simulink model "wingrockCustom"  (R2025b)
settings: Solver=VariableStepAuto  StartTime=0.0  StopTime=Tf  RelTol=1e-3
undefined symbols (not defined in the file): A, B
libraries: slctrl_adaptive x1
settings Model: Creator=The MathWorks, Inc.  LastModifiedBy=The MathWorks, Inc.
settings SolverCC: MaxZcPerStep=1.0
settings DebuggingCC: UnconnectedInputMsg=warning  UnconnectedOutputMsg=warning  UnconnectedLineMsg=warning
settings ModelReferenceCC: EnableRefExpFcnMdlSchedulingChecks=on
settings RTWCC: GPUComputeCapability=3.5  DLArmComputeVersion=19.05

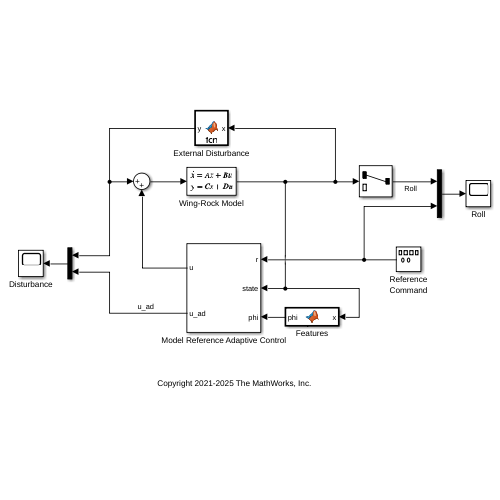
[thumbnail: Simulink's stored preview of the top-level diagram]
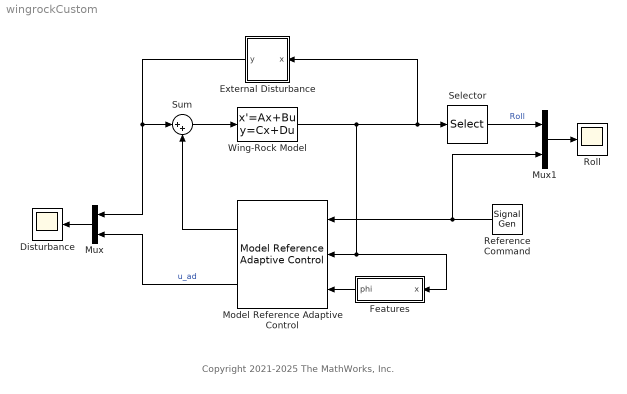
== system wingrockCustom ==
  note: Copyright 2021-2025 The MathWorks, Inc.
  Disturbance : Scope
      settings: ActiveDisplayYMinimum=-4.33702  ActiveDisplayYMaximum=6.96023
  External Disturbance : MATLAB Function  TreatAsAtomicUnit=on
  Features : MATLAB Function  TreatAsAtomicUnit=on
  Model Reference Adaptive Control : slctrl_adaptive/Model Reference Adaptive Control  selectType=Direct  A=A  B=B  Ahat=0  ALrEnable=on  gamma_a=1  ALrEnableMod=on  Bhat=1  BLrEnable=on  gamma_b=1  BLrEnableMod=on  externalKtauEnable=off  k_tau=-1  estParamOutput=off  Am=Am  Bm=Bm  kx=Kx  FBLrEnable=off  gamma_kx=1  FBLrEnableMod=on  kr=Kr  FFLrEnable=off  gamma_kr=1  FFLrEnableMod=on  AdaptEnable=on  gamma=gamma_w  WLrEnableMod=off  Q=Q  FeatureTypeOptions=Use External Source for Feature  shlHiddenLayerSize=10  gamma_V=0.1  nCen=N  cSpanMin=cen_min  cSpanMax=cen_max  cSig=bandwidth  adaptiveCntrlOutport=on  modChoice=None  sigma_val=0.1  DiscreteEnable=off  Ts=0.05  IntegrationMethods=Forward Euler
      settings: LibrarySourceBlock=slctrlblks/Adaptive Control/Model Reference Adaptive Control
  Mux : Mux  Inputs=2
  Mux1 : Mux  Inputs=2
  Reference Command : SignalGenerator  WaveForm=square  Frequency=0.5  Units=rad/sec
  Roll : Scope
      settings: ActiveDisplayYMinimum=-1.67014  ActiveDisplayYMaximum=1.67336
  Selector : Selector  InputPortWidth=2  IndexOptions=Index vector (dialog)  Indices=1  OutputSizes=1
  Sum : Sum  Inputs=|++
  Wing-Rock Model : StateSpace  A=[0 1;0 0]  B=[0;1]  C=eye(2)  D=[0;0]  InitialCondition=0
  wires:
  Reference Command/1 -> Model Reference Adaptive Control/1, Mux1/2
  Sum/1 -> Wing-Rock Model/1
  External Disturbance/1(y) -> Sum/1, Mux/1
  Model Reference Adaptive Control/1 -> Sum/2
  Wing-Rock Model/1 -> Selector/1, External Disturbance/1(x), Features/1(x), Model Reference Adaptive Control/2
  Mux/1 -> Disturbance/1
  Selector/1 -> Mux1/1  "Roll"
  Mux1/1 -> Roll/1
  Model Reference Adaptive Control/2 -> Mux/2  "u_ad"
  Features/1(phi) -> Model Reference Adaptive Control/3

== matlab function wingrockCustom/External Disturbance ==
  data: y output; x input
function y = fcn(x)

phi = [1 x(1) x(2) abs(x(1))*x(2) abs(x(2))*x(2) x(1)^3];

w = [1 0.2314 0.6918 0.6245 0.1 0.214];

u = w*phi';

y = u;

== matlab function wingrockCustom/Features ==
  data: x input; phi output
function phi = fcn(x)

phi = [1 x(1) x(2) abs(x(1))*x(2) abs(x(2))*x(2) x(1)^3]';
